simulink model "junyakaiguangai5"  (Simulink 8.8)
settings: Solver=ode4  StartTime=0.0  StopTime=inf  FixedStep=0.001  RelTol=1e-3  EnableMultiTasking=on
undefined symbols (not defined in the file or in its folder): mdaadlink6208, sigbuilder_block
libraries: xpcobsoletelib x24, slrtlib x2, simulink x1
(part 3 of 3)

== stateflow chart jinjichuli/jinjichuli ==
  state MANUAL
    state fa4_4 [parallel]
      settings: executionOrder=1
      state A
        entry:diancifa20=0;
      state on
        entry:diancifa20=1;
      (default) -> MANUAL.fa4_4.A
      MANUAL.fa4_4.on -> MANUAL.fa4_4.A : [fa20==0]
      MANUAL.fa4_4.A -> MANUAL.fa4_4.on : [fa20==1]
    state fa4_2 [parallel]
      settings: executionOrder=2
      state A
        entry:diancifa11_2=0;
      state on
        entry:diancifa11_2=1;
      (default) -> MANUAL.fa4_2.A
      MANUAL.fa4_2.on -> MANUAL.fa4_2.A : [fa11_2==0]
      MANUAL.fa4_2.A -> MANUAL.fa4_2.on : [fa11_2==1]
    state fa4_3 [parallel]
      settings: executionOrder=3
      state A
        entry:diancifa11_5=0;
      state on
        entry:diancifa11_5=1;
      (default) -> MANUAL.fa4_3.A
      MANUAL.fa4_3.on -> MANUAL.fa4_3.A : [fa11_5==0]
      MANUAL.fa4_3.A -> MANUAL.fa4_3.on : [fa11_5==1]
    state fa4_1 [parallel]
      settings: executionOrder=4
      state A
        entry:diancifa11_1=0;
      state on
        entry:diancifa11_1=1;
      (default) -> MANUAL.fa4_1.A
      MANUAL.fa4_1.on -> MANUAL.fa4_1.A : [fa11_1==0]
      MANUAL.fa4_1.A -> MANUAL.fa4_1.on : [fa11_1==1]
    state fa4_5 [parallel]
      settings: executionOrder=5
      state A
        entry:diancifa16_1=0;
      state on
        entry:diancifa16_1=1;
      (default) -> MANUAL.fa4_5.A
      MANUAL.fa4_5.on -> MANUAL.fa4_5.A : [fa16_1==0]
      MANUAL.fa4_5.A -> MANUAL.fa4_5.on : [fa16_1==1]
    state fa4_6 [parallel]
      settings: executionOrder=6
      state A
        entry:diancifa3=0;
      state on
        entry:diancifa3=1;
      (default) -> MANUAL.fa4_6.A
      MANUAL.fa4_6.on -> MANUAL.fa4_6.A : [fa3==0]
      MANUAL.fa4_6.A -> MANUAL.fa4_6.on : [fa3==1]
    state fa4_8 [parallel]
      settings: executionOrder=7
      state A
        entry:xuansong=0;
      state on
        entry:xuansong=1;
      (default) -> MANUAL.fa4_8.A
      MANUAL.fa4_8.on -> MANUAL.fa4_8.A : [xuansongmingling==0]
      MANUAL.fa4_8.A -> MANUAL.fa4_8.on : [xuansongmingling==1]
    state fa4_7 [parallel]
      settings: executionOrder=8
      state A
        entry:diancifa21=0;
      state on
        entry:diancifa21=1;
      (default) -> MANUAL.fa4_7.A
      MANUAL.fa4_7.on -> MANUAL.fa4_7.A : [fa21==0]
      MANUAL.fa4_7.A -> MANUAL.fa4_7.on : [fa21==1]
    state fa4_9 [parallel]
      settings: executionOrder=9
      state A
        entry:xuanjin=0;
      state on
        entry:xuanjin=1;
      (default) -> MANUAL.fa4_9.A
      MANUAL.fa4_9.on -> MANUAL.fa4_9.A : [xuanjinmingling==0]
      MANUAL.fa4_9.A -> MANUAL.fa4_9.on : [xuanjinmingling==1]
    state fa4_10 [parallel]
      settings: executionOrder=10
      state A
        entry:suoding=0;
      state on
        entry:suoding=1;
      (default) -> MANUAL.fa4_10.A
      MANUAL.fa4_10.on -> MANUAL.fa4_10.A : [suodingmingling==0]
      MANUAL.fa4_10.A -> MANUAL.fa4_10.on : [suodingmingling==1]
    state fa4_12 [parallel]
      settings: executionOrder=11
      state A
        entry:bililiuliangfa18_1=0;
      state on
        entry:bililiuliangfa18_1=1;
      (default) -> MANUAL.fa4_12.A
      MANUAL.fa4_12.on -> MANUAL.fa4_12.A : [fa18_1==0]
      MANUAL.fa4_12.A -> MANUAL.fa4_12.on : [fa18_1==1]
    state fa4_11 [parallel]
      settings: executionOrder=12
      state A
        entry:jiesuo=0;
      state on
        entry:jiesuo=1;
      (default) -> MANUAL.fa4_11.A
      MANUAL.fa4_11.on -> MANUAL.fa4_11.A : [jiesuomingling==0]
      MANUAL.fa4_11.A -> MANUAL.fa4_11.on : [jiesuomingling==1]
    state fa4_13 [parallel]
      settings: executionOrder=13
      state A
        entry:bililiuliangfa18_2=0;
      state on
        entry:bililiuliangfa18_2=1;
      (default) -> MANUAL.fa4_13.A
      MANUAL.fa4_13.on -> MANUAL.fa4_13.A : [fa18_2==0]
      MANUAL.fa4_13.A -> MANUAL.fa4_13.on : [fa18_2==1]
    state kiagai [parallel]
      settings: executionOrder=14
      state A
        entry:bililiuliangfa18_3=0;
      state on
        entry:bililiuliangfa18_3=1;
      (default) -> MANUAL.kiagai.A
      MANUAL.kiagai.on -> MANUAL.kiagai.A : [fa18_3==0]
      MANUAL.kiagai.A -> MANUAL.kiagai.on : [fa18_3==1]
    state yajin [parallel]
      settings: executionOrder=15
      state A
        entry:bililiuliangfa18_4=0;
      state on
        entry:bililiuliangfa18_4=1;
      (default) -> MANUAL.yajin.A
      MANUAL.yajin.on -> MANUAL.yajin.A : [fa18_4==0]
      MANUAL.yajin.A -> MANUAL.yajin.on : [fa18_4==1]
    state kaigai [parallel]
      settings: executionOrder=16
      state A
        entry:kaiguangaifa=0;
      state on
        entry:kaiguangaifa=1;
      (default) -> MANUAL.kaigai.A
      MANUAL.kaigai.on -> MANUAL.kaigai.A : [fa_kgg==0]
      MANUAL.kaigai.A -> MANUAL.kaigai.on : [fa_kgg==1]
  state off1
  state on1
    entry:
    diancifa11_1=0;
    diancifa11_2=0;
    diancifa11_5=0;
    diancifa20=0;
    diancifa16_1=0;
    diancifa3=0;
    diancifa21=0;
    xuansong=0;
    xuanjin=0;
    suoding=0;
    jiesuo=0;
    bililiuliangfa18_1=0;
    bililiuliangfa18_2=0;
    bililiuliangfa18_3=0;
    bililiuliangfa18_4=0;
    kaiguangaifa=0;
  state end
    en:
    diancifa11_1=0;
    diancifa11_2=0;
    diancifa11_5=0;
    diancifa20=0;
    diancifa16_1=0;
    diancifa3=0;
    diancifa21=0;
    xuansong=0;
    xuanjin=0;
    suoding=0;
    jiesuo=0;
    bililiuliangfa18_1=0;
    bililiuliangfa18_2=0;
    bililiuliangfa18_3=0;
    bililiuliangfa18_4=0;
    kaiguangaifa=0;
  (default) -> off1
  off1 -> on1 : [reset==1]
  on1 -> MANUAL : after(5000,tick)
  MANUAL -> end : [jieshu==1]
  data: reset input double; diancifa11_1 output double; diancifa11_2 output double; diancifa11_5 output double; diancifa20 output double; diancifa16_1 output double; diancifa3 output double; diancifa21 output double; suoding output double; jiesuo output double; xuansong output double; xuanjin output double; bililiuliangfa18_1 output double; bililiuliangfa18_2 output double; fa11_1 input double; fa11_2 input double; fa11_5 input double; fa20 input double; fa16_1 input double; fa3 input double; fa21 input double; suodingmingling input double; jiesuomingling input double; xuansongmingling input double; xuanjinmingling input double; fa18_1 input double; fa18_2 input double; bililiuliangfa18_3 output double; bililiuliangfa18_4 output double; kaiguangaifa output double; fa18_3 input double; fa18_4 input double; fa_kgg input double; jieshu input double

== stateflow chart Subsystem2/shoudong/Chart ==
  state shoudong
    state SXQxieya [parallel]
      settings: executionOrder=1
      state off1
        entry:
        diancifa11_1=0;
        bililiuliangfa18_3=0;
        bililiuliangfa18_4=0;
      state on1
        entry:
        diancifa11_5=1;
      state xieya1
        entry:
        bililiuliangfa18_1=1;
        bililiuliangfa18_2=1;
        p0_2=p0sheding;
      state xieya1_2
        entry:
        bililiuliangfa18_1=1;
        bililiuliangfa18_2=0;
      state xieya1_1
        entry:
        bililiuliangfa18_1=1;
        bililiuliangfa18_2=1;
      state xieya1_3
        entry:
        bililiuliangfa18_1=0;
        bililiuliangfa18_2=1;
      state xieya2
        entry:
        bililiuliangfa18_1=1;
        bililiuliangfa18_2=1;
        p0_2=p0_2-0.03;
      state xieya7_2
        entry:
        bililiuliangfa18_1=1;
        bililiuliangfa18_2=0;
      state xieya7_1
        entry:
        bililiuliangfa18_1=1;
        bililiuliangfa18_2=1;
      state xieya7_3
        entry:
        bililiuliangfa18_1=0;
        bililiuliangfa18_2=1;
      state off2
        entry:
        diancifa11_5=0;
        bililiuliangfa18_1=0;
        bililiuliangfa18_2=0;
        SXQxieyawancheng=1;
      state xieya8
        entry:
        diancifa11_5=1;
        bililiuliangfa18_1=1;
        bililiuliangfa18_2=1;
      (default) -> shoudong.SXQxieya.off1
      shoudong.SXQxieya.off1 -> shoudong.SXQxieya.on1 : [SXQxieya==1]
      shoudong.SXQxieya.on1 -> xieya1 : after(500,tick)
      xieya1 -> (junction 525)
      (junction 525) -> xieya1_2 [order 2] : [p2<=p0_2&&p3>p0_2]
      (junction 525) -> xieya1_1 [order 1] : [p2>p0_2&&p3>p0_2]
      xieya1_2 -> (junction 525)
      xieya1_3 -> (junction 525)
      xieya1_1 -> (junction 525)
      (junction 525) -> xieya1_3 [order 3] : [p2>p0_2&&p3<=p0_2]
      (junction 525) -> xieya2 [order 4] : [p2<=p0_2&&p3<=p0_2]
      (junction 526) -> (junction 525) [order 2] : [p0_2>p0_0]
      xieya2 -> (junction 526)
      (junction 526) -> (junction 527) [order 1] : [p0_2<=p0_0]
      (junction 527) -> xieya7_2 [order 2] : [p2<=p0_0&&p3>p0_0]
      xieya7_2 -> (junction 527)
      (junction 527) -> xieya7_1 [order 1] : [p2>p0_0&&p3>p0_0]
      xieya7_3 -> (junction 527)
      (junction 527) -> xieya7_3 [order 3] : [p2>p0_0&&p3<=p0_0]
      xieya7_1 -> (junction 527)
      (junction 527) -> xieya8 [order 4] : [p2<=p0_0&&p3<=p0_0]
      (junction 528) -> (junction 527) [order 2] : [p2>p0_0||p3>p0_0]
      (junction 528) -> shoudong.SXQxieya.off2 [order 1] : [p2<=p0_0&&p3<=p0_0]
      xieya8 -> (junction 528) : after(3000,tick)
    state kaiguangai [parallel]
      settings: executionOrder=2
      state start
        entry:
        xuansong=0;
        xuanjin=0;
        suoding=0;
        jiesuo=0;
        kaigaikaishi=0;
        guangaikaishi=0;
        diancifa20=0;
      state on5
        entry:
        jiesuo=1;
      state off5
        entry:
        jiesuo=0;
      state on1
        entry:diancifa20=1;
      state on6
        entry:
        guangaikaishi=1;
      state on2
        entry:
        xuansong=1;
      state on7
        entry:
        guangaikaishi=0;
      state off1
        entry:
        xuansong=0;
      state on71
        entry:
        diancifa20=1;
      state off2
        entry:
        diancifa20=0;
        SQshiyabuchangwancheng=1;
      state on8
        entry:
        xuanjin=1;
      state off6
        entry:
        xuanjin=0;
      state on3
        entry:
        kaigaikaishi=1;
      state on4
        entry:
        kaigaikaishi=0;
      state off7
        entry:
        diancifa20=0;
        SQxuanjinjianyawancheng=1;
        guangaiwancheng=1;
      state on41
        entry:
        suoding=1;
      state off3
        entry:
        suoding=0;
      state off4
        entry:
        kaigaiwancheng=1;
      (default) -> shoudong.kaiguangai.start
      shoudong.kaiguangai.off4 -> on5 : [jiesuomingling==1]
      on5 -> shoudong.kaiguangai.off5 : [jiesuodaowei1==1&&jiesuodaowei2==1]
      shoudong.kaiguangai.start -> shoudong.kaiguangai.on1 : [shiyabuchang==1]
      shoudong.kaiguangai.off5 -> on6 : after(1000,tick)[guangai==1]
      shoudong.kaiguangai.on1 -> shoudong.kaiguangai.on2 : [liuliangji==1&&p1==p2&&xuansongmingling==1]
      on6 -> on7 : [guangaijieshu==1]
      shoudong.kaiguangai.on2 -> shoudong.kaiguangai.off1 : [xuansongdaowei1==1&&xuansongdaowei2==1]
      on7 -> on71 : [xuanjinjianya==1]
      on71 -> on8 : [liuliangji==1&&p1==p2&&xuanjinmingling==1]
      shoudong.kaiguangai.off1 -> shoudong.kaiguangai.off2 : after(500,tick)
      on8 -> shoudong.kaiguangai.off6 : [xuanjindaowei1==1&&xuanjindaowei2==1]
      shoudong.kaiguangai.off2 -> shoudong.kaiguangai.on3 : after(1000,tick)[kaigai==1]
      shoudong.kaiguangai.off6 -> off7 : after(500,tick)
      shoudong.kaiguangai.on3 -> on4 : [kaigaijieshu==1]
      on4 -> on41 : [suodingmingling==1]
      on41 -> shoudong.kaiguangai.off3 : [suodingdaowei1==1&&suodingdaowei2==1]
      shoudong.kaiguangai.off3 -> shoudong.kaiguangai.off4 : after(500,tick)
    state SCjiaya [parallel]
      settings: executionOrder=3
      state off1
        entry:diancifa11_1=0;
        diancifa11_2=0;
        diancifa16_1=0;
      state on1
        entry:diancifa11_1=1;
        diancifa11_2=1;
        diancifa16_1=0;
      state off2
        entry:
        diancifa11_1=0;
        diancifa11_2=0;
        diancifa16_1=0;
      state on3
        entry:diancifa11_1=1;
        diancifa11_2=1;
        diancifa16_1=0;
      state on2
        entry:diancifa16_1=1;
      state off3
        entry:
        diancifa11_1=0;
        diancifa11_2=0;
        diancifa16_1=0;
      state off4
        entry:
        SCjiayawancheng=1;
      (default) -> shoudong.SCjiaya.off1
      shoudong.SCjiaya.off1 -> shoudong.SCjiaya.on1 : [SCjiaya==1]
      shoudong.SCjiaya.on1 -> shoudong.SCjiaya.off2 : [p1>=p1sheding-0.005]
      shoudong.SCjiaya.off2 -> (junction 571) : after(5000,tick)
      shoudong.SCjiaya.on2 -> (junction 571)
      shoudong.SCjiaya.on3 -> (junction 571)
      (junction 571) -> shoudong.SCjiaya.on2 [order 2] : [p1>p1sheding+0.005]
      (junction 571) -> shoudong.SCjiaya.on3 [order 1] : [p1<(p1sheding-0.005)]
      (junction 571) -> shoudong.SCjiaya.off3 [order 3] : [p1>=(p1sheding-0.005)&&p1<=p1sheding+0.005]
      shoudong.SCjiaya.off3 -> shoudong.SCjiaya.off4
    state SCzhushui [parallel]
      settings: executionOrder=4
      state off4
        entry:diancifa16_1=0;
        diancifa3=0;
      state on2
        entry:diancifa16_1=1;
      state on3
        entry:diancifa3=1;
      state off1
        entry:diancifa3=0;
      state off2
        entry:diancifa16_1=0;
      state off3
        entry:
        SCzhushuiwancheng=1;
      (default) -> shoudong.SCzhushui.off4
      shoudong.SCzhushui.off4 -> shoudong.SCzhushui.on2 : [SCzhushui==1]
      shoudong.SCzhushui.on2 -> shoudong.SCzhushui.on3 : after(20,tick)
      shoudong.SCzhushui.on3 -> shoudong.SCzhushui.off1 : [fuqiuyeweikongzhiqi==1]
      shoudong.SCzhushui.off1 -> shoudong.SCzhushui.off2
      shoudong.SCzhushui.off2 -> shoudong.SCzhushui.off3
    state SXQjunya [parallel]
      settings: executionOrder=5
      state jiaya1_1
        entry:
        bililiuliangfa18_3=1;
        bililiuliangfa18_4=1;
      state jiaya7_1
        entry:
        bililiuliangfa18_3=1;
        bililiuliangfa18_4=1;
      state jiaya2
        entry:
        bililiuliangfa18_3=1;
        bililiuliangfa18_4=1;
        p0_1=p0_1+0.03;
      state off1
        entry:
        diancifa20=0;
        bililiuliangfa18_1=0;
        bililiuliangfa18_2=0;
      state jiaya1
        entry:
        bililiuliangfa18_3=1;
        bililiuliangfa18_4=1;
        p0_1=p0_0;
      state on1
        entry:
        diancifa11_1=1;
        diancifa11_5=1;
      state off2
        entry:
        diancifa11_5=0;
        bililiuliangfa18_3=0;
        bililiuliangfa18_4=0;
      state jiance1_35
        entry:
        bililiuliangfa18_1=0;
        bililiuliangfa18_2=1;
      state jiance1_34
        entry:
        bililiuliangfa18_1=1;
        bililiuliangfa18_2=0;
      state jiaya7_3
        entry:
        bililiuliangfa18_3=0;
        bililiuliangfa18_4=1;
      state jiaya7_2
        entry:
        bililiuliangfa18_3=1;
        bililiuliangfa18_4=0;
      state jiaya1_2
        entry:
        bililiuliangfa18_3=1;
        bililiuliangfa18_4=0;
      state jiaya1_3
        entry:
        bililiuliangfa18_3=0;
        bililiuliangfa18_4=1;
      state jiance1_33
        entry:
        diancifa11_5=0;
      state jiance2_34
        entry:
        bililiuliangfa18_3=1;
        bililiuliangfa18_4=0;
      state jiance2_33
        entry:
        diancifa11_5=0;
      state jiance2_32
        entry:
        bililiuliangfa18_3=1;
        bililiuliangfa18_4=1;
      state jiance2_31
        entry:
        diancifa11_5=1;
      state jiance1_36
        entry:
        diancifa11_5=0;
        bililiuliangfa18_1=0;
        bililiuliangfa18_2=0;
      state jiance1_32
        entry:
        bililiuliangfa18_1=1;
        bililiuliangfa18_2=1;
      state jiance2_35
        entry:
        bililiuliangfa18_3=0;
        bililiuliangfa18_4=1;
      state off5
        entry:
        diancifa11_5=0;
        bililiuliangfa18_3=0;
        bililiuliangfa18_4=0;
      state jiance2_36
        entry:
        diancifa11_5=0;
        bililiuliangfa18_3=0;
        bililiuliangfa18_4=0;
      state jiance1_31
        entry:
        diancifa11_5=1;
      state off3
        entry:
        diancifa11_5=0;
        bililiuliangfa18_3=0;
        bililiuliangfa18_4=0;
      state off6
        entry:
        diancifa11_1=0;
        SXQjunyawancheng=1;
      state jiance1_21
        entry:
        bililiuliangfa18_1=1;
      state off4
        entry:
        diancifa11_5=0;
        bililiuliangfa18_3=0;
        bililiuliangfa18_4=0;
      state jiance1_22
        entry:
        bililiuliangfa18_1=0;
      state jiance1_11
        entry:
        diancifa11_5=1;
      state jiance1_14
        entry:
        bililiuliangfa18_2=0;
      state jiance2_11
        entry:
        diancifa11_5=1;
      state jiance2_14
        entry:
        bililiuliangfa18_4=0;
      state jiance2_21
        entry:
        bililiuliangfa18_3=1;
      state jiance1_12
        entry:
        bililiuliangfa18_2=1;
      state jiance1_13
        entry:
        diancifa11_5=0;
      state jiance2_22
        entry:
        bililiuliangfa18_3=0;
      state jiance2_12
        entry:
        bililiuliangfa18_4=1;
      state jiance2_13
        entry:
        diancifa11_5=0;
      jiaya1_1 -> (junction 588)
      (junction 588) -> jiaya2 [order 4] : [p2>=p0_1&&p3>=p0_1]
      (junction 588) -> jiaya1_1 [order 1] : [p2<p0_1&&p3<p0_1]
      jiaya7_1 -> (junction 590)
      (junction 590) -> jiaya7_1 [order 1] : [p2<p0sheding&&p3<p0sheding]
      (default) -> shoudong.SXQjunya.off1
      jiaya2 -> (junction 589)
      (junction 590) -> shoudong.SXQjunya.off2 [order 4] : [p2>=p0sheding&&p3>=p0sheding]
      jiaya1 -> (junction 588)
      (junction 589) -> (junction 588) [order 2] : [p0_1<p0sheding]
      (junction 589) -> (junction 590) [order 1] : [p0_1>=p0sheding]
      (junction 588) -> jiaya1_3 [order 3] : [p2<p0_1&&p3>=p0_1]
      shoudong.SXQjunya.on1 -> jiaya1 : after(500,tick)
      shoudong.SXQjunya.off1 -> shoudong.SXQjunya.on1 : [SXQjunya==1]
      jiaya1_3 -> (junction 588)
      (junction 590) -> jiaya7_2 [order 2] : [p2>=p0sheding&&p3<p0sheding]
      (junction 590) -> jiaya7_3 [order 3] : [p2<p0sheding&&p3>=p0sheding]
      jiaya7_3 -> (junction 590)
      jiaya7_2 -> (junction 590)
      (junction 588) -> jiaya1_2 [order 2] : [p2>=p0_1&&p3<p0_1]
      jiaya1_2 -> (junction 588)
      jiance1_35 -> (junction 591)
      shoudong.SXQjunya.off2 -> (junction 594) : after(3000,tick)
      jiance1_34 -> (junction 591)
      (junction 591) -> jiance1_35 [order 2] : [p2>(p0sheding+0.012)&&p3<=(p0sheding+0.012)]
      jiance1_33 -> jiance1_34
      jiance2_33 -> jiance2_34
      (junction 591) -> jiance1_33 [order 1] : [p2<=(p0sheding+0.012)&&p3>(p0sheding+0.012)]
      (junction 591) -> jiance1_36 [order 3] : [p2<=(p0sheding+0.012)&&p3<=(p0sheding+0.012)]
      jiance1_32 -> (junction 591)
      jiance2_32 -> (junction 592)
      (junction 592) -> jiance2_33 [order 1] : [p2>=(p0sheding-0.01)&&p3<(p0sheding-0.001)]
      jiance2_34 -> (junction 592)
      jiance2_31 -> jiance2_32
      (junction 592) -> jiance2_35 [order 2] : [p2<(p0sheding-0.01)&&p3>=(p0sheding-0.001)]
      jiance2_35 -> (junction 592)
      (junction 592) -> jiance2_36 [order 3] : [p2>=(p0sheding-0.01)&&p3>=(p0sheding-0.001)]
      (junction 596) -> jiance2_31 [order 5] : [p2<(p0sheding-0.01)&&p3<(p0sheding-0.001)]
      jiance1_31 -> jiance1_32
      jiance1_36 -> (junction 594)
      (junction 594) -> jiance1_31 [order 3] : [p2>(p0sheding+0.012)&&p3>(p0sheding+0.012)]
      (junction 596) -> shoudong.SXQjunya.off5 [order 1] : [p2>=(p0sheding-0.01)&&p2<=(p0sheding+0.012)&&p3>=(p0sheding-0.01)&&p3<=(p0sheding+0.012)]
      shoudong.SXQjunya.off3 -> (junction 593) : after(1000,tick)
      (junction 593) -> (junction 596) [order 1] : [p2<=(p0sheding+0.012)&&p3<=(p0sheding+0.012)]
      (junction 594) -> shoudong.SXQjunya.off3 [order 4] : [p2<=(p0sheding+0.012)&&p3<=(p0sheding+0.012)]
      (junction 593) -> (junction 594) [order 2] : [p2>(p0sheding+0.012)||p3>(p0sheding+0.012)]
      shoudong.SXQjunya.off5 -> (junction 595) : after(1000,tick)
      jiance2_36 -> (junction 596)
      (junction 594) -> jiance1_21 [order 2] : [p2<=(p0sheding+0.012)&&p3>(p0sheding+0.012)]
      (junction 597) -> (junction 596) [order 2] : [p2<=(p0sheding+0.012)&&p3<=(p0sheding+0.012)]
      (junction 597) -> (junction 594) [order 1] : [p2>(p0sheding+0.012)||p3>(p0sheding+0.012)]
      jiance1_22 -> (junction 594)
      jiance1_14 -> (junction 594)
      (junction 594) -> jiance1_11 [order 1] : [p2>(p0sheding+0.012)&&p3<=(p0sheding+0.012)]
      (junction 595) -> (junction 596) [order 2] : [p2<(p0sheding-0.01)||p2>(p0sheding+0.012)||p3<(p0sheding-0.01)||p3>(p0sheding+0.012)]
      (junction 595) -> shoudong.SXQjunya.off6 [order 1] : [p2>=(p0sheding-0.01)&&p2<=(p0sheding+0.012)&&p3>=(p0sheding-0.01)&&p3<=(p0sheding+0.012)]
      (junction 596) -> shoudong.SXQjunya.off4 [order 2] : [p2>(p0sheding+0.012)||p3>(p0sheding+0.012)]
      (junction 596) -> jiance2_21 [order 4] : [p2>=(p0sheding-0.01)&&p3<(p0sheding-0.001)]
      jiance2_14 -> (junction 596)
      jiance2_22 -> (junction 596)
      (junction 596) -> jiance2_11 [order 3] : [p2<(p0sheding-0.01)&&p3>=(p0sheding-0.001)]
      jiance1_21 -> jiance1_22 : [p2<=(p0sheding+0.012)&&p3<=(p0sheding+0.012)]
      shoudong.SXQjunya.off4 -> (junction 597) : after(1000,tick)
      jiance1_11 -> jiance1_12
      jiance1_13 -> jiance1_14
      jiance2_11 -> jiance2_12
      jiance2_13 -> jiance2_14
      jiance2_21 -> jiance2_22 : [p2>=(p0sheding-0.01)&&p3>=(p0sheding-0.001)]
      jiance1_12 -> jiance1_13 : [p2<=(p0sheding+0.012)&&p3<=(p0sheding+0.012)]
      jiance2_12 -> jiance2_13 : [p2>=(p0sheding-0.01)&&p3>=(p0sheding-0.001)]
  state start
    en:
    diancifa11_1=0;
    diancifa11_2=0;
    diancifa11_5=0;
    diancifa20=0
    diancifa16_1=0;
    diancifa3=0;
    diancifa21=0;
    bililiuliangfa18_1=0;
    bililiuliangfa18_2=0;
    bililiuliangfa18_3=0;
    bililiuliangfa18_4=0;
    xuansong=0;
    xuanjin=0;
    suoding=0;
    jiesuo=0;
    kaigaikaishi=0;
    guangaikaishi=0;
  state off111
    en:
    diancifa11_1=0;
    diancifa11_2=0;
    diancifa11_5=0;
    diancifa20=0
    diancifa16_1=0;
    diancifa3=0;
    diancifa21=0;
    bililiuliangfa18_1=0;
    bililiuliangfa18_2=0;
    bililiuliangfa18_3=0;
    bililiuliangfa18_4=0;
    xuansong=0;
    xuanjin=0;
    suoding=0;
    jiesuo=0;
    SCzhushuiwancheng=0;
    SCjiayawancheng=0;
    SXQjunyawancheng=0;
    SQshiyabuchangwancheng=0;
    kaigaikaishi=0;
    kaigaiwancheng=0;
    SQxuanjinjianyawancheng=0;
    guangaikaishi=0;
    guangaiwancheng=0;
    SXQxieyawancheng=0;
  (default) -> start
  start -> shoudong : [start==1]
  shoudong -> off111 : [jieshu==1]
  data: start input double; diancifa11_1 output double; diancifa11_2 output double; diancifa11_5 output double; SCzhushui input double; fuqiuyeweikongzhiqi input double; diancifa20 output double; diancifa16_1 output double; diancifa3 output double; SCjiaya input double; SXQjunya input double; diancifa21 output double; suoding output double; jiesuo output double; xuansong output double; xuanjin output double; bililiuliangfa18_1 output double; bililiuliangfa18_2 output double; bililiuliangfa18_3 output double; bililiuliangfa18_4 output double; SXQxieya input double; p1 input double; p1sheding input double; liuliangji input double; p2 input double; p3 input double; p0_0 input double; p0sheding input double; kaigaikaishi output double; guangaikaishi output double; SCzhushuiwancheng output double; SCjiayawancheng output double; SXQjunyawancheng output double; SXQxieyawancheng output double; SQshiyabuchangwancheng output double; SQxuanjinjianyawancheng output double; kaigaiwancheng output double; guangaiwancheng output double; xuansongdaowei1 input double; xuansongdaowei2 input double; xuanjindaowei1 input double; xuanjindaowei2 input double; suodingdaowei1 input double; suodingdaowei2 input double; jiesuodaowei1 input double; jiesuodaowei2 input double; kaigaijieshu input double; guangaijieshu input double; p0_1 local double; p0_2 local double; jieshu input double; kaigai input double; guangai input double; shiyabuchang input double; xuansongmingling input double; suodingmingling input double; jiesuomingling input double; xuanjinjianya input double; xuanjinmingling input double
